simulink model "simulation"  (R2021b)
settings: Solver=ode4  StartTime=0.0  StopTime=10  FixedStep=Ts  RelTol=1e-3  EnableMultiTasking=on
undefined symbols (not defined in the file or in its folder): q0dot, q10, q20
settings Model: Creator=giusepp  LastModifiedBy=Rita
settings SolverCC: AlgebraicLoopSolver=TrustRegion
settings DataIOCC: LimitDataPoints=on  SaveFormat=Array  ReturnWorkspaceOutputs=off
settings OptimizationCC: LifeSpan=inf
settings DebuggingCC: SolverPrmCheckMsg=warning  SFUnexpectedBacktrackingDiag=warning  SFNoUnconditionalDefaultTransitionDiag=warning  SFExecutionAtInitializationDiag=none  SFMachineParentedDataDiag=warning  ArithmeticOperatorsInVariantConditions=warning
settings HardwareCC: ProdBitPerPointer=32  ProdBitPerSizeT=32  ProdBitPerPtrDiffT=32  ProdLargestAtomicFloat=None  ProdIntDivRoundTo=Undefined  ProdEndianess=Unspecified  ProdWordSize=32  ProdHWDeviceType=32-bit Generic
settings ModelReferenceCC: PropagateSignalLabelsOutOfModel=off
settings SFSimCC: SimUseLocalCustomCode=off  CustomCodeUndefinedFunction=UseInterfaceOnly
settings RTWCC: RTWUseLocalCustomCode=off
settings CodeAppCC: StateflowObjectComments=on
settings GRTTargetCC: TargetLangStandard=C89/C90 (ANSI)
settings ConfigComp: CovMetricSettings=dw  CovSaveCumulativeToWorkspaceVar=on  CovSaveSingleToWorkspaceVar=on  CovExternalEMLEnable=off  CovSFcnEnable=off

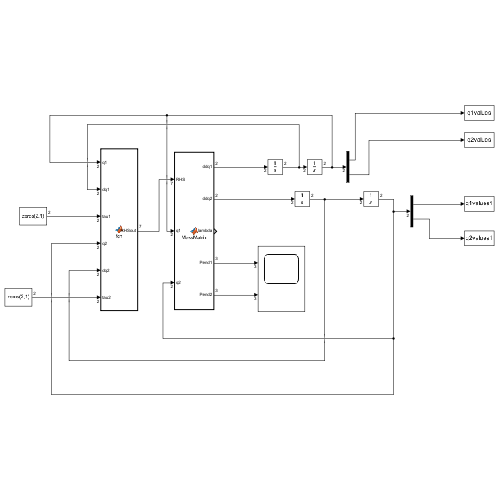
[thumbnail: Simulink's stored preview of the top-level diagram]
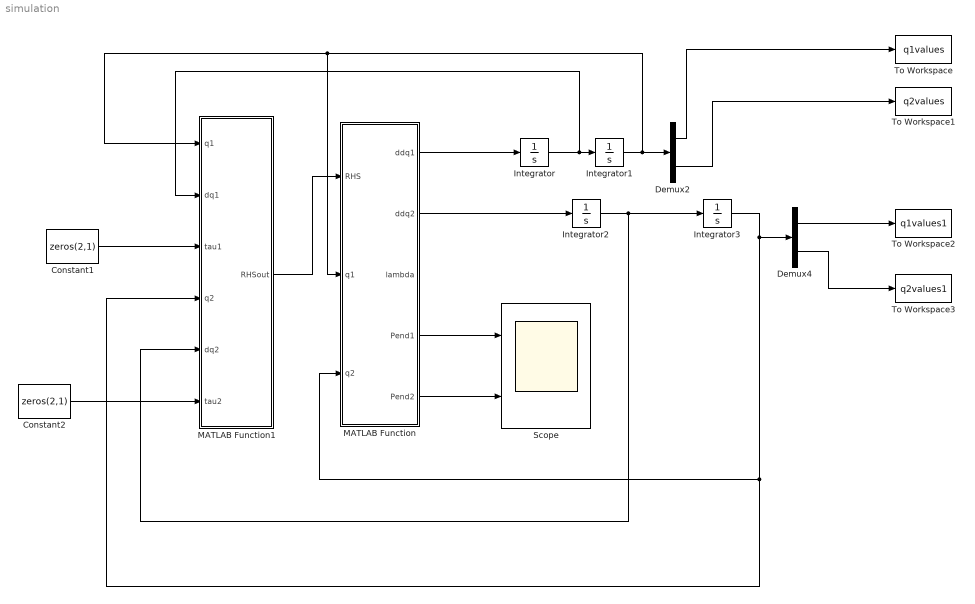
== system simulation ==
  Constant1 : Constant  Value=zeros(2,1)
  Constant2 : Constant  Value=zeros(2,1)
  Demux2 : Demux  Outputs=2
  Demux4 : Demux  Outputs=2
  Integrator : Integrator  InitialCondition=q0dot
  Integrator1 : Integrator  InitialCondition=q10
  Integrator2 : Integrator  InitialCondition=q0dot
  Integrator3 : Integrator  InitialCondition=q20
  MATLAB Function : MATLAB Function  TreatAsAtomicUnit=on
  MATLAB Function1 : MATLAB Function  TreatAsAtomicUnit=on
  Scope : Scope  NumInputPorts=2
  To Workspace : ToWorkspace  VariableName=q1values  SaveFormat=Timeseries  SampleTime=-1
  To Workspace1 : ToWorkspace  VariableName=q2values  SaveFormat=Timeseries  SampleTime=-1
  To Workspace2 : ToWorkspace  VariableName=q1values1  SaveFormat=Timeseries  SampleTime=-1
  To Workspace3 : ToWorkspace  VariableName=q2values1  SaveFormat=Timeseries  SampleTime=-1
  wires:
  Integrator/1 -> Integrator1/1, MATLAB Function1/2(dq1)
  Integrator1/1 -> Demux2/1, MATLAB Function1/1(q1), MATLAB Function/2(q1)
  Demux2/1 -> To Workspace/1
  Demux2/2 -> To Workspace1/1
  MATLAB Function1/1(RHSout) -> MATLAB Function/1(RHS)
  Constant1/1 -> MATLAB Function1/3(tau1)
  Integrator2/1 -> Integrator3/1, MATLAB Function1/5(dq2)
  Integrator3/1 -> MATLAB Function/3(q2), MATLAB Function1/4(q2), Demux4/1
  Constant2/1 -> MATLAB Function1/6(tau2)
  Demux4/1 -> To Workspace2/1
  Demux4/2 -> To Workspace3/1
  MATLAB Function/2(ddq2) -> Integrator2/1
  MATLAB Function/1(ddq1) -> Integrator/1
  MATLAB Function/4(Pend1) -> Scope/1
  MATLAB Function/5(Pend2) -> Scope/2

== matlab function simulation/MATLAB Function1 ==
  data: q1 input; RHSout output; dq1 input; tau1 input; q2 input; dq2 input; tau2 input
function RHSout = fcn(q1,dq1,tau1,q2,dq2,tau2)

RHSout = RHS(q1,dq1,tau1,q2,dq2,tau2);

== matlab function simulation/MATLAB Function ==
  data: RHS input; q1 input; ddq1 output; ddq2 output; lambda output; q2 input; Pend1 output; Pend2 output
function [ddq1,ddq2,lambda,Pend1,Pend2] = MassMatrix(RHS,q1,q2)

IM = modifiedInertiaMatrix(q1,q2);

ddQ = IM\RHS;

Pend1 = Pend(q1);
Pend2 = Pend(q2);

ddq1 = ddQ(1:2);
ddq2 = ddQ(3:4);
lambda = ddQ(5:7);
